simulink model "RLC_circuit_ss"  (R2020b)
settings: Solver=VariableStepAuto  StartTime=0.0  StopTime=3  RelTol=1e-3
settings Model: Creator=kjartan  LastModifiedBy=kjartan

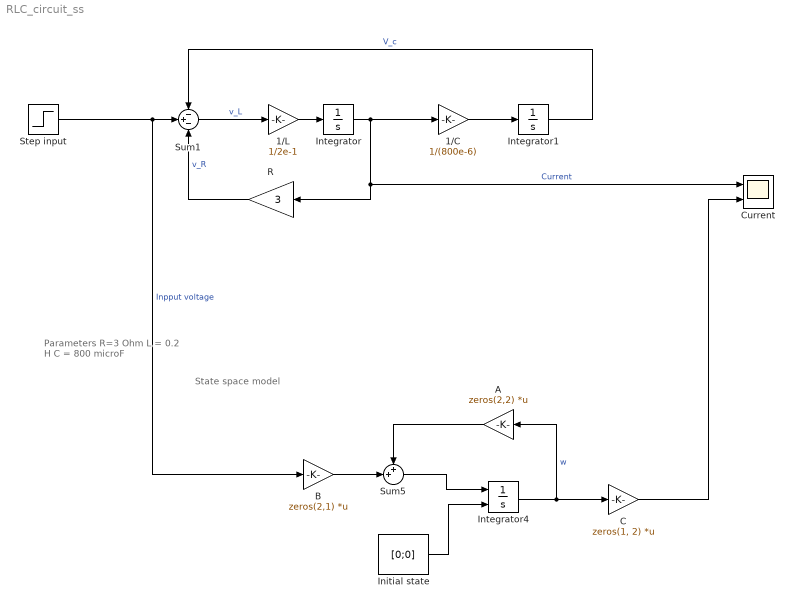
== system RLC_circuit_ss ==
  note: Parameters
      |
      | R=3 Ohm
      | L = 0.2 H
      | C = 800 microF
  note: State space model
  1/C : Gain  Gain=1/(800e-6)
  1/L : Gain  Gain=1/2e-1
  A : Gain  Gain=zeros(2,2)  Multiplication=Matrix(K*u) (u vector)
  B : Gain  Gain=zeros(2,1)  Multiplication=Matrix(K*u)
  C : Gain  Gain=zeros(1, 2)  Multiplication=Matrix(K*u) (u vector)
  Current : Scope  NumInputPorts=2
  Initial state : Constant  Value=[0;0]
  Integrator : Integrator
  Integrator1 : Integrator
  Integrator4 : Integrator  InitialConditionSource=external
  R : Gain  Gain=3
  Step input : Step  Time=0  After=20  SampleTime=0
  Sum1 : Sum  Inputs=-+-
  Sum5 : Sum  Inputs=++|
  wires:
  Integrator1/1 -> Sum1/1  "V_c"
  Integrator/1 -> R/1, Current/1, 1/C/1  "Current"
  1/L/1 -> Integrator/1
  R/1 -> Sum1/3  "v_R"
  Sum1/1 -> 1/L/1  "v_L"
  Step input/1 -> B/1, Sum1/2  "Inpput voltage"
  1/C/1 -> Integrator1/1
  Integrator4/1 -> A/1, C/1  "w"
  Sum5/1 -> Integrator4/1
  Initial state/1 -> Integrator4/2
  B/1 -> Sum5/2
  A/1 -> Sum5/1
  C/1 -> Current/2
